simulink model "simulink1"  (R2016a)
settings: Solver=VariableStepAuto  StartTime=0.0  StopTime=10.0  RelTol=1e-3
values from neighbouring files (symbols this model uses):
  g = 9.81    [pendulum.m]
  H = 0.100    (= 0.1)    [pendulum.m]
  L = 1.0    (= 1)    [pendulum.m]
  rho = 3000.0    (= 3000)    [pendulum.m]
  theta0 = -pi/2    (= -1.57079632679)    [pendulum.m]
  v0 = 0    [pendulum.m]
  W = 0.100    (= 0.1)    [pendulum.m]
undefined symbols (not defined in the file or in its folder): magnitude
settings Model: Creator=simone  LastModifiedBy=simone

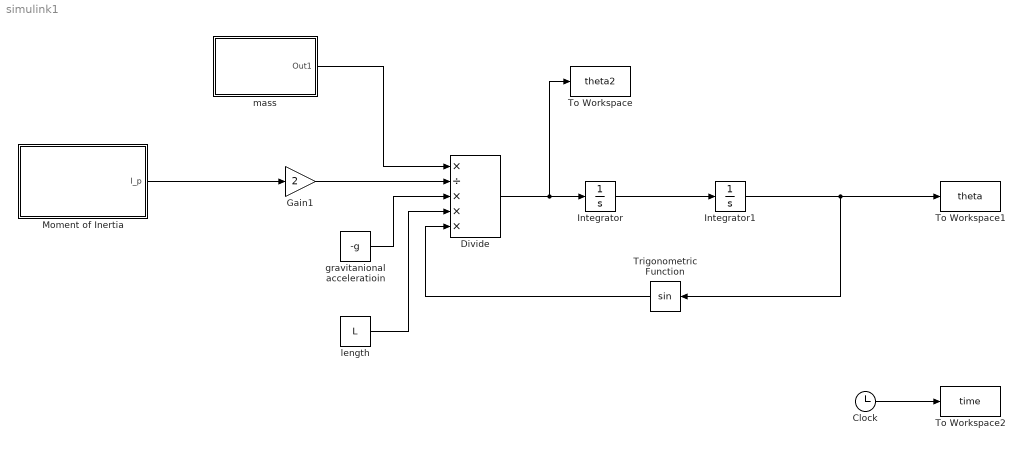
== system simulink1 ==
  Clock : Clock
  Divide : Product  Inputs=*/***
  Gain1 : Gain  Gain=2
  Integrator : Integrator  InitialCondition=v0
  Integrator1 : Integrator  InitialCondition=theta0
  Moment of Inertia : Subsystem
  To Workspace : ToWorkspace  VariableName=theta2  SaveFormat=Timeseries  SampleTime=-1
  To Workspace1 : ToWorkspace  VariableName=theta  SaveFormat=Timeseries  SampleTime=-1
  To Workspace2 : ToWorkspace  VariableName=time  SaveFormat=Timeseries  SampleTime=-1
  Trigonometric Function : Trigonometry
  gravitanional acceleratioin : Constant  Value=-g
  length : Constant  Value=L
  "mass " : Subsystem
  wires:
  Integrator/1 -> Integrator1/1
  Integrator1/1 -> Trigonometric Function/1, To Workspace1/1
  gravitanional acceleratioin/1 -> Divide/3
  length/1 -> Divide/4
  Trigonometric Function/1 -> Divide/5
  Clock/1 -> To Workspace2/1
  "mass "/1(Out1) -> Divide/1
  Gain1/1 -> Divide/2
  Divide/1 -> To Workspace/1, Integrator/1
  Moment of Inertia/1("I_p ") -> Gain1/1

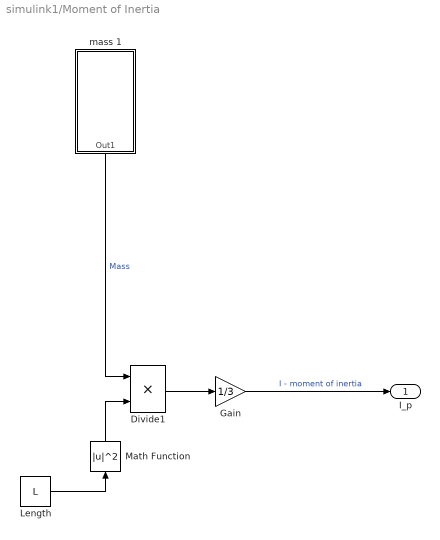
== system simulink1/Moment of Inertia ==
  Divide1 : Product  Inputs=**
  Gain : Gain  Gain=1/3
  Length : Constant  Value=L
  Math Function : Math  Operator=magnitude^2  SaturateOnIntegerOverflow=on
  mass 1 : Subsystem
  "I_p " : Outport
  wires:
  Gain/1 -> "I_p "/1  "I - moment of inertia"
  mass 1/1(Out1) -> Divide1/1  "Mass"
  Divide1/1 -> Gain/1
  Math Function/1 -> Divide1/2
  Length/1 -> Math Function/1

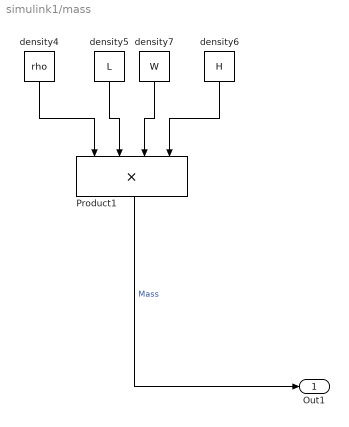
== system simulink1/mass  ==
  Product1 : Product  Inputs=4
  density4 : Constant  Value=rho
  density5 : Constant  Value=L
  density6 : Constant  Value=H
  density7 : Constant  Value=W
  Out1 : Outport
  wires:
  Product1/1 -> Out1/1  "Mass"
  density7/1 -> Product1/3
  density6/1 -> Product1/4
  density4/1 -> Product1/1
  density5/1 -> Product1/2

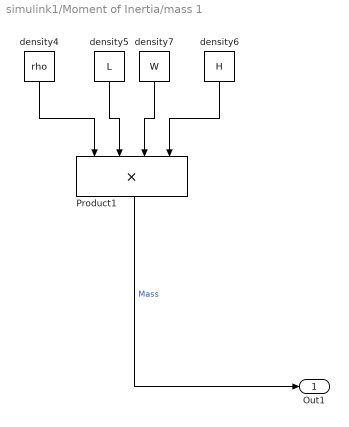
== system simulink1/Moment of Inertia/mass 1 ==
  Product1 : Product  Inputs=4
  density4 : Constant  Value=rho
  density5 : Constant  Value=L
  density6 : Constant  Value=H
  density7 : Constant  Value=W
  Out1 : Outport
  wires:
  Product1/1 -> Out1/1  "Mass"
  density7/1 -> Product1/3
  density6/1 -> Product1/4
  density4/1 -> Product1/1
  density5/1 -> Product1/2
